simulink model "Experiment_AERO_pitch_channel"  (Simulink 8.9)
settings: Solver=ode4  StartTime=0.0  StopTime=100  FixedStep=0.001  RelTol=1e-3  EnableMultiTasking=on
InitFcn:
  | Parameters_and_initial_conditions
values from neighbouring files (symbols this model uses):
  A_p = [0 1 ... (first row only)    [Parameters_and_initial_conditions.m]
  B_p = [0 ... (first row only)    [Parameters_and_initial_conditions.m]
  C_p = [1 0;0 1]    [Parameters_and_initial_conditions.m]
  D_p = [0;0]    [Parameters_and_initial_conditions.m]
  Dp = 0.007768621416960    (= 0.00776862141696)    [Parameters_and_initial_conditions.m]
  Dp_static = Dp*0.05    (= 0.000388431070848)    [Parameters_and_initial_conditions.m]
  Dy = 0.0220    (= 0.022)    [Parameters_and_initial_conditions.m]
  G_bar_D = [(Jp*T^2) (T^2*Dp+2*Jp*T) (T^2*Ksp+2*T*Dp+T*k2+Jp) (2*T*Ksp+T*k1+Dp+k2) (Ksp+k1)]    [Parameters_and_initial_conditions.m]
  G_bar_N11 = [(Jp*T) (T*Dp+Jp) (T*Ksp+Dp+k2) Ksp]    [Parameters_and_initial_conditions.m]
  G_bar_N12 = [-k2]    [Parameters_and_initial_conditions.m]
  G_bar_N21 = [-k1 0]    [Parameters_and_initial_conditions.m]
  G_bar_N22 = [(Jp*T) (T*Dp+Jp) (T*Ksp+Dp) (Ksp+k1)]    [Parameters_and_initial_conditions.m]
  Invalid_T = 1    [Parameters_and_initial_conditions.m]
  Jp = J_body + 2*J_prop    (= 0.0218868648283)    [Parameters_and_initial_conditions.m]
  Jy = J_body + 2*J_prop + J_yoke    (= 0.0219920648283)    [Parameters_and_initial_conditions.m]
  k1 = 0.1    [Parameters_and_initial_conditions.m]
  k2 = 0.05    [Parameters_and_initial_conditions.m]
  Kpp = 9.971955650940002e-04    (= 0.000997195565094)    [Parameters_and_initial_conditions.m]
  Kpy = 0.0021    [Parameters_and_initial_conditions.m]
  Ksp = 0.071643279410402    (= 0.0716432794104)    [Parameters_and_initial_conditions.m]
  Kyp = -0.0027    [Parameters_and_initial_conditions.m]
  Kyy = 0.0022    [Parameters_and_initial_conditions.m]
  PitchAxisEnable = 1    [Parameters_and_initial_conditions.m]
  PitchMotorEnable = 1    [Parameters_and_initial_conditions.m]
  psi_dot_initial = 0.0    (= 0)    [Parameters_and_initial_conditions.m]
  psi_initial = 0.0    (= 0)    [Parameters_and_initial_conditions.m]
  T = 2    [Parameters_and_initial_conditions.m]
  theta_dot_initial = 0.0    (= 0)    [Parameters_and_initial_conditions.m]
  theta_initial = 0.0    (= 0)    [Parameters_and_initial_conditions.m]
  YawAxisEnable = 0    [Parameters_and_initial_conditions.m]
  YawMotorEnable = 0    [Parameters_and_initial_conditions.m]
undefined symbols (not defined in the file or in its folder): Continuous, Time
libraries: simulink_extras x11, quarc_library x9, ctrlSharedLib x1, quanser_aero x1
settings Model: Creator=MLevis  LastModifiedBy=fsc  SimulationMode=external  ExtModeTrigDuration=5000
settings SolverCC: PositivePriorityOrder=on
settings DataIOCC: SignalLoggingSaveFormat=Dataset
settings DebuggingCC: UnderspecifiedInitializationDetection=Simplified  MergeDetectMultiDrivingBlocksExec=error  SolverPrmCheckMsg=warning  FcnCallInpInsideContextMsg=error  StateNameClashWarn=none
settings RTWCC: SystemTargetFile=quarc_win64.tlc  TemplateMakefile=quarc_default_tmf  Description=QUARC Win64 Target
settings STFCustomTargetCC: TargetPreCompLibLocation=C:\PROGRA~3\QUARC\lib\2017a\win64\release  ConcurrentExecutionCompliant=on  GeneratePreprocessorConditionals=Disable all  SystemTargetFile=quarc_win64.tlc
settings GRTTargetCC: TargetPreCompLibLocation=C:\PROGRA~3\QUARC\lib\2017a\win64\release  ParMdlRefBuildCompliant=off  CompOptLevelCompliant=off  MatFileLogging=off  CPPClassGenCompliant=off  UseToolchainInfoCompliant=off  ExtMode=on  ExtModeMexFile=quarc_comm
settings ConfigComp: CovSFcnEnable=off

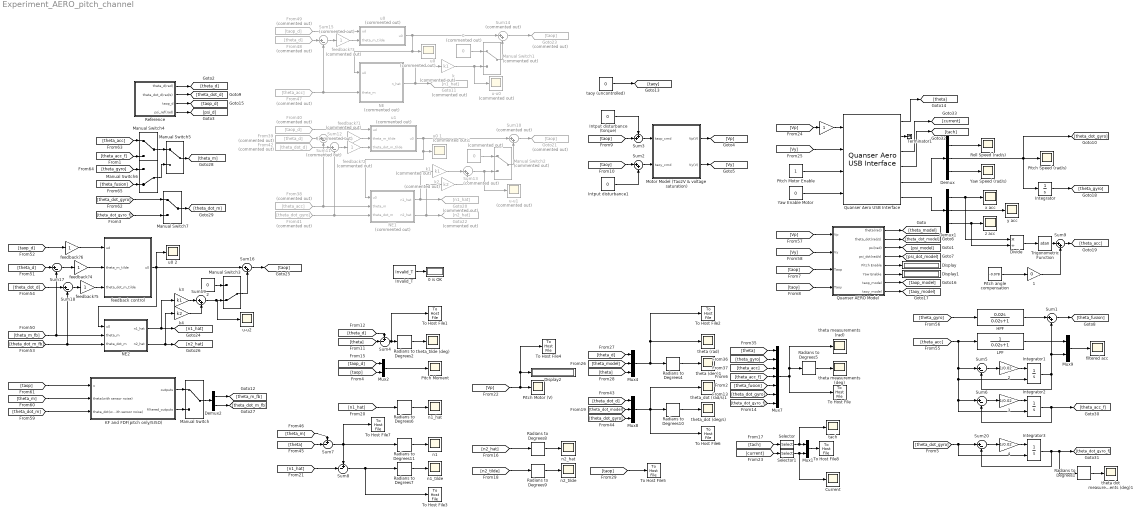
== system Experiment_AERO_pitch_channel ==
  " " : Gain
  " 1" : Gain  Gain=0
  " 2" : Gain  Gain=1/0.02
  " 3" : Gain  Gain=1/0.02
  " 4" : Gain  Gain=1/0.02
  " feedback?1" : Gain  Commented=on
  " feedback?2" : Gain  Commented=on
  " feedback?3" : Gain  Commented=on
  " feedback?4" : Gain
  " feedback?5" : Gain
  " feedback?6" : Gain
  0 : Constant  Commented=on  Value=0
  0 is OK : Display
  1 : Constant  Commented=on  Value=0
  2 : Constant  Value=0
  Current : Scope
  Demux : Demux  Outputs=3
  Demux1 : Demux  Outputs=3
  Demux2 : Demux  Outputs=2
  Display : Display
  Display1 : Display
  Display2 : Display
  Divide : Product  Inputs=*/
  From38 : From  Commented=on  GotoTag=theta_acc
  From39 : From  Commented=on  GotoTag=theta_d
  From40 : From  Commented=on  GotoTag=taop_d
  From41 : From  Commented=on  GotoTag=theta_dot_gyro
  From42 : From  Commented=on  GotoTag=theta_dot_d
  From47 : From  Commented=on  GotoTag=theta_acc
  From48 : From  Commented=on  GotoTag=theta_d
  From49 : From  Commented=on  GotoTag=taop_d
  Goto11 : Goto  Commented=on  GotoTag=n1_hat
  Goto20 : Goto  Commented=on  GotoTag=n1_hat
  Goto21 : Goto  Commented=on  GotoTag=taop
  Goto22 : Goto  Commented=on  GotoTag=n2_hat
  Goto23 : Goto  Commented=on  GotoTag=taop
  HPF : TransferFcn  Numerator=[0.02 0]  Denominator=[0.02 1]
  Integrator : Integrator
  Integrator1 : Integrator  InitialConditionSource=external
  Integrator2 : Integrator  InitialConditionSource=external
  Integrator3 : Integrator  InitialConditionSource=external
  Intput disturbance (torque) : Constant  Value=0
  Intput disturbance1 : Constant  Value=0
  Invalid_T : Constant  Value=Invalid_T
  KF and FDF(pitch only/SISO) : Subsystem
  LPF : TransferFcn  Denominator=[0.02 1]
  Manual Switch{,4..5,7} (4 alike) : ManualSwitch
  Manual Switch1 : ManualSwitch  Commented=on
  Manual Switch2 : ManualSwitch  Commented=on
  Manual Switch3 : ManualSwitch  CurrentSetting=0
  Manual Switch6 : ManualSwitch  CurrentSetting=0
  Motor Model (Tao2V & voltage saturation) : Subsystem
  Mux1 : Mux  Inputs=2
  Mux2 : Mux  Inputs=2
  Mux4 : Mux  Inputs=3
  Mux7 : Mux  Inputs=7
  Mux8 : Mux  Inputs=3
  Mux9 : Mux  Inputs=2
  NE : Subsystem  Commented=on
  NE1 : Subsystem  Commented=on
  NE2 : Subsystem
  Pitch Moment : Scope
  Pitch Motor (V) : Scope
  Pitch Motor Enable : Constant
  Pitch Speed (rad/s) : Scope
  Pitch angle compensation : Constant  Value=-0.078
  Quanser AERO Model : Subsystem
  Quanser Aero USB Interface : quanser_aero/Quanser Aero USB Interface
  Radians to Degrees{1..2,4..11} (10 alike) : simulink_extras/Transformations/Radians to Degrees
  Reference : Subsystem
  Roll Speed (rad/s) : Scope
  Selector : Selector  InputPortWidth=2  IndexOptions=Index vector (dialog)  Indices=[1]  OutputSizes=1
  Selector1 : Selector  InputPortWidth=2  IndexOptions=Index vector (dialog)  Indices=[1]  OutputSizes=1
  Sum{1..2,9,16,19} (5 alike) : Sum  Inputs=|++
  Sum10 : Sum  Commented=on  Inputs=|++
  Sum11 : Sum  Commented=on  Inputs=|+-
  Sum12 : Sum  Commented=on  Inputs=|+-
  Sum13 : Sum  Commented=on  Inputs=|++
  Sum14 : Sum  Commented=on  Inputs=|++
  Sum15 : Sum  Commented=on  Inputs=|+-
  Sum{5..6,17..18,20} (5 alike) : Sum  Inputs=|+-
  Sum3 : Sum  Inputs=++|
  Sum4 : Sum  Inputs=+-|
  Sum7 : Sum  Inputs=+-|
  Sum8 : Sum  Inputs=+-|
  Terminator1 : Terminator
  To Host File : quarc_library/Sinks/To Host/To Host File  file_name=Log_Sensor_Measurements.mat  variable_name=Log_Sensor_Measurements  decimation=1  sample_time=-1  file_format=MAT-file v.5  options=No header or footer  append=off  final_file_name=Log_Sensor_Measurements.mat  bitrate=2000000
  To Host File1 : quarc_library/Sinks/To Host/To Host File  file_name=Log_Tracking_Err.mat  variable_name=Log_Tracking_Err  decimation=1  sample_time=-1  file_format=MAT-file v.5  options=No header or footer  append=off  final_file_name=Log_Tracking_Err.mat  bitrate=2000000
  To Host File2 : quarc_library/Sinks/To Host/To Host File  file_name=Log_Theta_Response.mat  variable_name=Log_Theta_Response  decimation=1  sample_time=-1  file_format=MAT-file v.5  options=No header or footer  append=off  final_file_name=Log_Theta_Response.mat  bitrate=2000000
  To Host File3 : quarc_library/Sinks/To Host/To Host File  file_name=Log_Noise_Estimation_Err.mat  variable_name=Log_Noise_Estimation_Err  decimation=1  sample_time=-1  file_format=MAT-file v.5  options=No header or footer  append=off  final_file_name=Log_Noise_Estimation_Err.mat  bitrate=2000000
  To Host File4 : quarc_library/Sinks/To Host/To Host File  file_name=Log_Input_Voltage.mat  variable_name=Log_Input_Voltage  decimation=1  sample_time=-1  file_format=MAT-file v.5  options=No header or footer  append=off  final_file_name=Log_Input_Voltage.mat  bitrate=2000000
  To Host File5 : quarc_library/Sinks/To Host/To Host File  file_name=Log_Input_Torque.mat  variable_name=Log_Input_Torque  decimation=1  sample_time=-1  file_format=MAT-file v.5  options=No header or footer  append=off  final_file_name=Log_Input_Torque.mat  bitrate=2000000
  To Host File6 : quarc_library/Sinks/To Host/To Host File  file_name=Log_Theta_dot_Response.mat  variable_name=Log_Theta_dot_Response  decimation=1  sample_time=-1  file_format=MAT-file v.5  options=No header or footer  append=off  final_file_name=Log_Theta_dot_Response.mat  bitrate=2000000
  To Host File7 : quarc_library/Sinks/To Host/To Host File  file_name=Log_Noise.mat  variable_name=Log_Noise  decimation=1  sample_time=-1  file_format=MAT-file v.5  options=No header or footer  append=off  final_file_name=Log_Noise.mat  bitrate=2000000
  To Host File8 : quarc_library/Sinks/To Host/To Host File  file_name=Log_Tach_Current.mat  variable_name=Log_Tach_Current  decimation=1  sample_time=-1  file_format=MAT-file v.5  options=No header or footer  append=off  final_file_name=Log_Tach_Current.mat  bitrate=2000000
  Trigonometric Function : Trigonometry  Operator=atan
  Yaw Enable Motor : Constant  Value=0
  Yaw Speed (rad/s) : Scope
  feedback control : Subsystem
  filtered acc : Scope
  k : Gain  Commented=on  Gain=k1
  k1 : Gain  Commented=on  Gain=k1
  k2 : Gain  Commented=on  Gain=k2
  k3 : Gain  Gain=k1
  k4 : Gain  Gain=k2
  n1 : Scope
  n1_hat : Scope
  n1_tilde : Scope
  n2_hat : Scope
  n2_tilde : Scope
  tach : Scope
  taoy (uncontrolled) : Constant  Value=0
  theta (deg)1 : Scope
  theta (rad) : Scope
  theta dot measurements (deg)1 : Scope
  theta measurements (deg) : Scope
  theta measurements (rad) : Scope
  theta_dot (deg/s) : Scope
  theta_dot (rad/s)1 : Scope
  theta_tilde (deg) : Scope
  u-u0 : Scope  Commented=on
  u-u1 : Scope  Commented=on
  u-u2 : Scope
  u0 : Subsystem  Commented=on
  "u0 " : Scope  Commented=on
  u0 1 : Scope  Commented=on
  u0 2 : Scope
  u1 : Subsystem  Commented=on
  x acc : Scope
  y acc : Scope
  z acc : Scope
  wires:
  Quanser AERO Model/3(psi(rad)) -> [psi_model]
  Quanser AERO Model/1(theta(rad)) -> [theta_model]
  Reference/1(theta_d(rad)) -> [theta_d]
  Reference/4(psi_ref(rad)) -> [psi_d]
  Mux2/1 -> Pitch Moment/1
  Quanser AERO Model/2(theta_dot(rad/s)) -> [theta_dot_model]
  Quanser AERO Model/4(psi_dot(rad/s)) -> [psi_dot_model]
  Quanser AERO Model/5(Pitch Enable) -> Display/1
  Quanser AERO Model/6(Yaw Enable) -> Display1/1
  Motor Model (Tao2V & voltage saturation)/1(Vp(V)) -> [Vp]
  Motor Model (Tao2V & voltage saturation)/2(Vy(V)) -> [Vy]
  [taop] -> Sum3/2
  [taoy] -> Sum2/1
  Intput disturbance (torque)/1 -> Sum3/1
  Sum2/1 -> Motor Model (Tao2V & voltage saturation)/2(taoy_cmd)
  Sum3/1 -> Motor Model (Tao2V & voltage saturation)/1(taop_cmd)
  Intput disturbance1/1 -> Sum2/2
  [theta_d] -> Sum4/1
  [theta] -> Sum4/2
  Sum4/1 -> To Host File1/1, Radians to Degrees2/1
  Radians to Degrees2/1 -> theta_tilde (deg)/1
  Reference/2(theta_dot_d(rad/s)) -> [theta_dot_d]
  Reference/3(taop_d) -> [taop_d]
  [taop] -> Mux2/2
  [taop_d] -> Mux2/1
  Invalid_T/1 -> 0 is OK/1
  taoy (uncontrolled)/1 -> [taoy]
  [Vp] -> To Host File4/1, Display2/1, Pitch Motor (V)/1
  Quanser Aero USB Interface/5 -> Demux/1
  Yaw Enable Motor/1 -> Quanser Aero USB Interface/4
  Quanser Aero USB Interface/4 -> [tach]
  [Vp] -> " "/1
  Quanser Aero USB Interface/1 -> [theta]
  Demux/3 -> Yaw Speed (rad/s)/1
  Pitch Motor Enable/1 -> Quanser Aero USB Interface/3
  Quanser Aero USB Interface/3 -> [current]
  [Vy] -> Quanser Aero USB Interface/2
  Demux/1 -> Roll Speed (rad/s)/1
  Demux/2 -> [theta_dot_gyro], Integrator/1, Pitch Speed (rad/s)/1
  Quanser Aero USB Interface/2 -> Terminator1/1
  Quanser Aero USB Interface/6 -> Demux1/1
  " "/1 -> Quanser Aero USB Interface/1
  Radians to Degrees4/1 -> theta (deg)1/1
  [theta_model] -> Mux4/2
  [theta_d] -> Mux4/1
  [theta] -> Mux4/3
  Quanser AERO Model/7(taop_model) -> [taop_model]
  [taop] -> To Host File5/1
  Quanser AERO Model/8(taoy_model) -> [taoy_model]
  Integrator/1 -> [theta_gyro]
  [theta] -> Mux7/1
  Demux1/1 -> Divide/1, x acc/1
  Demux1/2 -> y acc/1
  Demux1/3 -> Divide/2, z acc/1
  Divide/1 -> Trigonometric Function/1
  Trigonometric Function/1 -> Sum9/1
  Sum9/1 -> [theta_acc]
  Pitch angle compensation/1 -> " 1"/1
  [theta_gyro] -> Mux7/2
  [theta_acc] -> Mux7/3
  Radians to Degrees5/1 -> theta measurements (deg)/1
  Manual Switch2/1 -> Sum10/2
  Sum11/1 -> " feedback?1"/1
  u1/1(u0) -> Sum10/1, NE1/1(u0), u0 1/1
  k1/1 -> Sum13/1
  NE1/1(n1_hat) -> Goto20/1, k1/1
  From39/1 -> Sum11/1
  Sum13/1 -> u-u1/1, Manual Switch2/2
  From40/1 -> u1/1(ud)
  From41/1 -> Sum12/2, NE1/3(theta_dot_m)
  k2/1 -> Sum13/2
  Sum12/1 -> " feedback?2"/1
  NE1/2(n2_hat) -> k2/1, Goto22/1
  Sum10/1 -> Goto21/1
  From38/1 -> Sum11/2, NE1/2(theta_m)
  1/1 -> Manual Switch2/1
  From42/1 -> Sum12/1
  " feedback?1"/1 -> u1/2(theta_m_tilde)
  " feedback?2"/1 -> u1/3(theta_dot_m_tilde)
  Sum8/1 -> To Host File3/1, Radians to Degrees7/1
  Radians to Degrees9/1 -> n2_tilde/1
  Radians to Degrees6/1 -> n1_hat/1
  [n2_tilde] -> Radians to Degrees9/1
  Radians to Degrees8/1 -> n2_hat/1
  [n2_hat] -> Radians to Degrees8/1
  [n1_hat] -> Radians to Degrees6/1
  Radians to Degrees7/1 -> n1_tilde/1
  Radians to Degrees10/1 -> theta_dot (deg/s)/1
  [theta_dot_model] -> Mux8/2
  Mux8/1 -> To Host File6/1, theta_dot (rad/s)1/1, Radians to Degrees10/1
  [theta_dot_gyro] -> Mux8/3
  [theta_dot_d] -> Mux8/1
  [theta_m] -> Sum7/1
  [theta] -> Sum7/2
  Sum7/1 -> To Host File7/1, Sum8/1, Radians to Degrees11/1
  [n1_hat] -> Sum8/2
  Radians to Degrees11/1 -> n1/1
  " 1"/1 -> Sum9/2
  0/1 -> Manual Switch1/1
  From48/1 -> Sum15/1
  Sum15/1 -> " feedback?3"/1
  From49/1 -> u0/1(ud)
  Manual Switch1/1 -> Sum14/2
  Sum14/1 -> Goto23/1
  NE/1(n_hat) -> Goto11/1, k/1
  k/1 -> u-u0/1, Manual Switch1/2
  From47/1 -> Sum15/2, NE/2(theta_m)
  u0/1(u0) -> "u0 "/1, NE/1(u0), Sum14/1
  " feedback?3"/1 -> u0/2(theta_m_tilde)
  Sum16/1 -> [taop]
  [taop_d] -> " feedback?6"/1
  [theta_dot_m_fb] -> Sum18/2, NE2/3(theta_dot_m)
  [theta_m_fb] -> Sum17/2, NE2/2(theta_m)
  Manual Switch3/1 -> Sum16/2
  " feedback?5"/1 -> feedback control/3(theta_dot_m_tilde)
  Sum19/1 -> u-u2/1, Manual Switch3/2
  [theta_dot_d] -> Sum18/1
  Sum18/1 -> " feedback?5"/1
  feedback control/1(u0) -> NE2/1(u0), u0 2/1, Sum16/1
  [theta_d] -> Sum17/1
  NE2/1(n1_hat) -> [n1_hat], k3/1
  " feedback?4"/1 -> feedback control/2(theta_m_tilde)
  k3/1 -> Sum19/1
  NE2/2(n2_hat) -> k4/1, [n2_hat]
  2/1 -> Manual Switch3/1
  Sum17/1 -> " feedback?4"/1
  k4/1 -> Sum19/2
  [theta_gyro] -> HPF/1
  HPF/1 -> Sum1/1
  LPF/1 -> Mux9/1
  Sum1/1 -> [theta_fusion]
  [theta_acc_f] -> Mux7/4
  Mux7/1 -> theta measurements (rad)/1, Radians to Degrees5/1, To Host File/1
  Integrator1/1 -> Sum5/2, Sum1/2, Mux9/2
  Sum5/1 -> " 2"/1
  " 2"/1 -> Integrator1/1
  Mux9/1 -> filtered acc/1
  [taop] -> Quanser AERO Model/3(Taop)
  [taoy] -> Quanser AERO Model/4(Taoy)
  [Vp] -> Quanser AERO Model/1(Vp)
  [Vy] -> Quanser AERO Model/2(Vy)
  " feedback?6"/1 -> feedback control/1(ud)
  [theta_dot_m] -> KF and FDF(pitch only/SISO)/3(theta_dot(with sensor noise))
  Demux2/2 -> [theta_dot_m_fb]
  Demux2/1 -> [theta_m_fb]
  [taop] -> KF and FDF(pitch only/SISO)/1(u)
  KF and FDF(pitch only/SISO)/2(filtered_outputs) -> Manual Switch/2
  KF and FDF(pitch only/SISO)/1(outputs) -> Manual Switch/1
  Manual Switch/1 -> Demux2/1
  Manual Switch7/1 -> [theta_dot_m]
  [theta_acc] -> Manual Switch4/1
  [theta_gyro] -> Manual Switch6/1
  Manual Switch4/1 -> Manual Switch5/1
  Manual Switch5/1 -> [theta_m]
  [theta_fusion] -> Manual Switch6/2
  [theta_m] -> KF and FDF(pitch only/SISO)/2(theta(with sensor noise))
  Mux4/1 -> To Host File2/1, theta (rad)/1, Radians to Degrees4/1
  [theta_acc_f] -> Manual Switch4/2
  Manual Switch6/1 -> Manual Switch5/2
  Integrator2/1 -> Sum6/2, [theta_acc_f]
  " 3"/1 -> Integrator2/1
  Sum6/1 -> " 3"/1
  [theta_acc] -> Sum6/1, Integrator2/2, Integrator1/2, Sum5/1, LPF/1
  [theta_fusion] -> Mux7/5
  [theta_dot_gyro] -> Manual Switch7/1
  [theta_dot_gyro_f] -> Manual Switch7/2
  [theta_dot_gyro] -> Integrator3/2, Sum20/1
  Sum20/1 -> " 4"/1
  " 4"/1 -> Integrator3/1
  Integrator3/1 -> Radians to Degrees1/1, [theta_dot_gyro_f], Sum20/2
  Radians to Degrees1/1 -> theta dot measurements (deg)1/1
  [theta_dot_gyro] -> Mux7/6
  [theta_dot_gyro_f] -> Mux7/7
  [tach] -> Selector/1
  Mux1/1 -> To Host File8/1
  [current] -> Selector1/1
  Selector/1 -> tach/1, Mux1/1
  Selector1/1 -> Current/1, Mux1/2

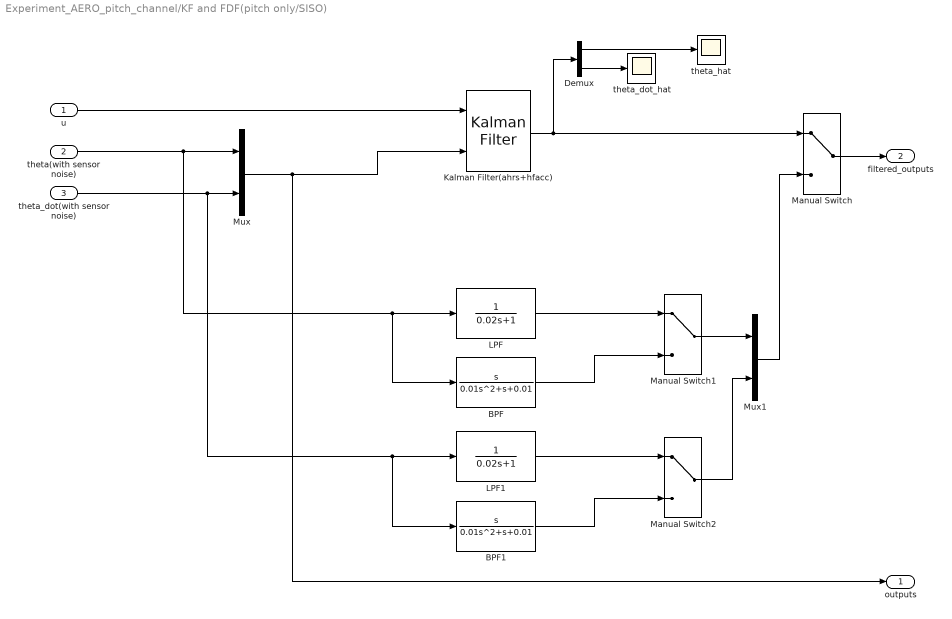
== system Experiment_AERO_pitch_channel/KF and FDF(pitch only/SISO) ==
  u : Inport
  theta(with sensor noise) : Inport  Port=2
  theta_dot(with sensor noise) : Inport  Port=3
  BPF : TransferFcn  Numerator=[1 0]  Denominator=[0.01 1 0.01]
  BPF1 : TransferFcn  Numerator=[1 0]  Denominator=[0.01 1 0.01]
  Demux : Demux  Outputs=2
  Kalman Filter(ahrs+hfacc) : ctrlSharedLib/Kalman Filter  TimeDomain=Continuous-Time  UseCurrentEstimator=on  ModelSource=Individual A, B, C, D matrices  ModelSourceVariable=ss(0.95,1,1,0,1)  A=A_p  B=B_p  C=C_p  D=D_p  NumberOfStates=1  NumberOfInputs=1  NumberOfOutputs=1  InitialEstimateSource=Dialog  X0=[theta_initial; theta_dot_initial]  P0=10  UseK=off  UseGH=off  NumberOfProcessNoiseInputs=1  G=1  TimeInvariantG=on  H=0  TimeInvariantH=on  Q=0.05*[1 0; 0 1]  TimeInvariantQ=on  R=[0.1 0.1]  TimeInvariantR=on  N=0  TimeInvariantN=on  AddInputPort=on  AddEnablePort=off  ExternalReset=none  OutputEstimatedY=off  OutputP=off  Ts=-1
  LPF : TransferFcn  Denominator=[0.02 1]
  LPF1 : TransferFcn  Denominator=[0.02 1]
  Manual Switch : ManualSwitch
  Manual Switch1 : ManualSwitch
  Manual Switch2 : ManualSwitch
  Mux : Mux  Inputs=2
  Mux1 : Mux  Inputs=2
  theta_dot_hat : Scope
  theta_hat : Scope
  outputs : Outport
  filtered_outputs : Outport  Port=2
  wires:
  Manual Switch/1 -> filtered_outputs/1
  u/1 -> Kalman Filter(ahrs+hfacc)/1
  Kalman Filter(ahrs+hfacc)/1 -> Demux/1, Manual Switch/1
  LPF/1 -> Manual Switch1/1
  theta(with sensor noise)/1 -> BPF/1, LPF/1, Mux/1
  BPF/1 -> Manual Switch1/2
  Demux/1 -> theta_hat/1
  Demux/2 -> theta_dot_hat/1
  Mux/1 -> outputs/1, Kalman Filter(ahrs+hfacc)/2
  LPF1/1 -> Manual Switch2/1
  theta_dot(with sensor noise)/1 -> LPF1/1, BPF1/1, Mux/2
  BPF1/1 -> Manual Switch2/2
  Manual Switch1/1 -> Mux1/1
  Manual Switch2/1 -> Mux1/2
  Mux1/1 -> Manual Switch/2

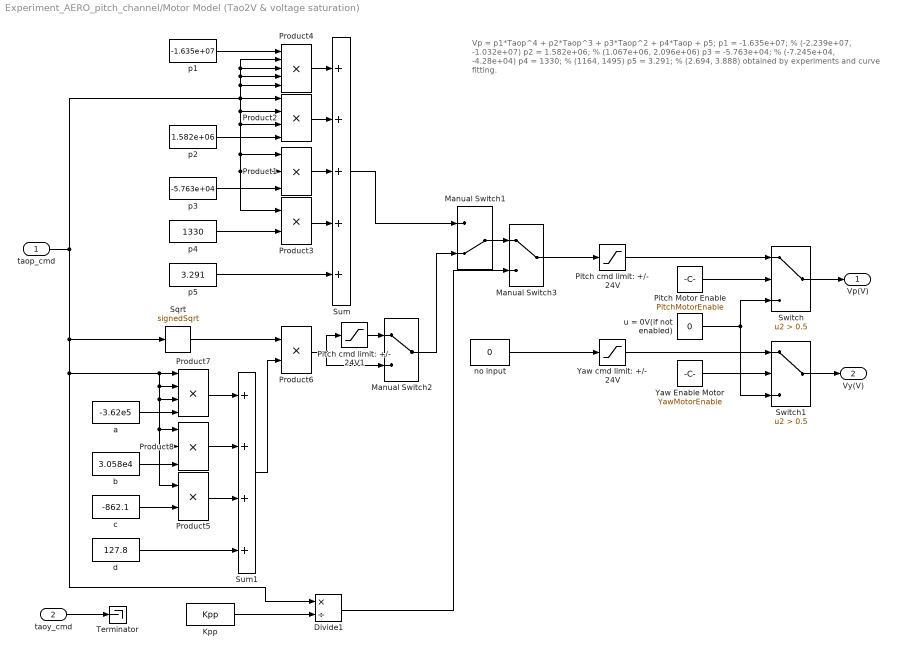
== system Experiment_AERO_pitch_channel/Motor Model (Tao2V & voltage saturation) ==
  note: Vp = p1*Taop^4 + p2*Taop^3 + p3*Taop^2 + p4*Taop + p5;
      | p1 = -1.635e+07; % (-2.239e+07, -1.032e+07)
      | p2 = 1.582e+06; % (1.067e+06, 2.096e+06)
      | p3 = -5.763e+04; % (-7.245e+04, -4.28e+04)
      | p4 = 1330; % (1164, 1495)
      | p5 = 3.291; % (2.694, 3.888)
      |
      | obtained by experiments and curve fitting.
  taop_cmd : Inport
  taoy_cmd : Inport  Port=2
  Divide1 : Product  Inputs=*/
  Kpp : Constant  Value=Kpp
  Manual Switch1 : ManualSwitch  CurrentSetting=0
  Manual Switch2 : ManualSwitch
  Manual Switch3 : ManualSwitch
  Pitch Motor Enable : Constant  Value=PitchMotorEnable
  Pitch cmd limit: +/- 24V : Saturate  UpperLimit=24  LowerLimit=-24
  Pitch cmd limit: +/- 24V1 : Saturate  UpperLimit=24  LowerLimit=0
  Product1 : Product  Inputs=3
  Product2 : Product  Inputs=4
  Product3 : Product
  Product4 : Product  Inputs=5
  Product5 : Product
  Product6 : Product
  Product7 : Product  Inputs=4
  Product8 : Product  Inputs=3
  Sqrt : Sqrt  Operator=signedSqrt  SaturateOnIntegerOverflow=on
  Sum : Sum  Inputs=+++++
  Sum1 : Sum  Inputs=++++
  Switch : Switch  Criteria=u2 > Threshold  Threshold=0.5
  Switch1 : Switch  Criteria=u2 > Threshold  Threshold=0.5
  Terminator : Terminator
  Yaw Enable Motor : Constant  Value=YawMotorEnable
  Yaw cmd limit: +/- 24V : Saturate  UpperLimit=24  LowerLimit=-24
  a : Constant  Value=-3.62e5
  b : Constant  Value=3.058e4
  c : Constant  Value=-862.1
  d : Constant  Value=127.8
  no input : Constant  Value=0
  p1 : Constant  Value=-1.635e+07
  p2 : Constant  Value=1.582e+06
  p3 : Constant  Value=-5.763e+04
  p4 : Constant  Value=1330
  p5 : Constant  Value=3.291
  u = 0V(if not enabled) : Constant  Value=0
  Vp(V) : Outport
  Vy(V) : Outport  Port=2
  wires:
  Pitch Motor Enable/1 -> Switch/2
  Yaw Enable Motor/1 -> Switch1/2
  Switch/1 -> Vp(V)/1
  Switch1/1 -> Vy(V)/1
  Yaw cmd limit: +/- 24V/1 -> Switch1/1
  Pitch cmd limit: +/- 24V/1 -> Switch/1
  u = 0V(if not enabled)/1 -> Switch1/3, Switch/3
  taoy_cmd/1 -> Terminator/1
  p2/1 -> Product2/4
  no input/1 -> Yaw cmd limit: +/- 24V/1
  Product2/1 -> Sum/2
  p3/1 -> Product1/3
  p4/1 -> Product3/2
  Kpp/1 -> Divide1/2
  Product1/1 -> Sum/3
  Product3/1 -> Sum/4
  p5/1 -> Sum/5
  Sum/1 -> Manual Switch1/1
  Product4/1 -> Sum/1
  p1/1 -> Product4/1
  Manual Switch3/1 -> Pitch cmd limit: +/- 24V/1
  a/1 -> Product7/4
  b/1 -> Product8/3
  Sum1/1 -> Product6/2
  Sqrt/1 -> Product6/1
  Product6/1 -> Pitch cmd limit: +/- 24V1/1, Manual Switch2/2
  Manual Switch1/1 -> Manual Switch3/1
  Divide1/1 -> Manual Switch3/2
  d/1 -> Sum1/4
  Product7/1 -> Sum1/1
  Product8/1 -> Sum1/2
  Product5/1 -> Sum1/3
  c/1 -> Product5/2
  taop_cmd/1 -> Sqrt/1, Divide1/1, Product7/1, Product7/2, Product7/3, Product8/1, Product8/2, Product5/1, Product4/5, Product4/4, Product4/3, Product4/2, Product2/1, Product3/1, Product1/2, Product1/1, Product2/3, Product2/2
  Pitch cmd limit: +/- 24V1/1 -> Manual Switch2/1
  Manual Switch2/1 -> Manual Switch1/2

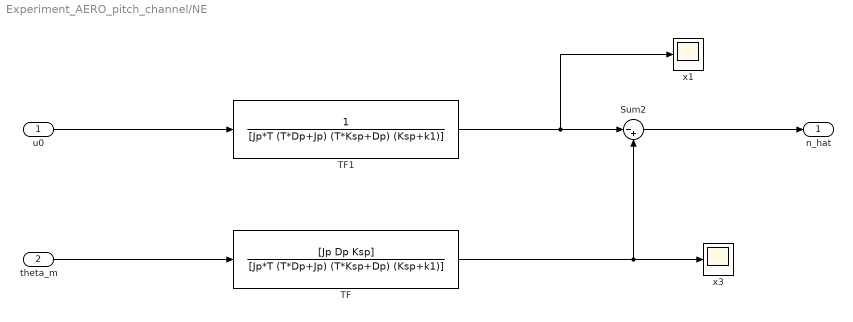
== system Experiment_AERO_pitch_channel/NE ==
  u0 : Inport
  theta_m : Inport  Port=2
  Sum2 : Sum  Inputs=|-+
  TF : TransferFcn  Numerator=[Jp Dp Ksp]  Denominator=[Jp*T (T*Dp+Jp) (T*Ksp+Dp) (Ksp+k1)]
  TF1 : TransferFcn  Denominator=[Jp*T (T*Dp+Jp) (T*Ksp+Dp) (Ksp+k1)]
  x1 : Scope
  x3 : Scope
  n_hat : Outport
  wires:
  theta_m/1 -> TF/1
  Sum2/1 -> n_hat/1
  TF/1 -> Sum2/2, x3/1
  u0/1 -> TF1/1
  TF1/1 -> x1/1, Sum2/1

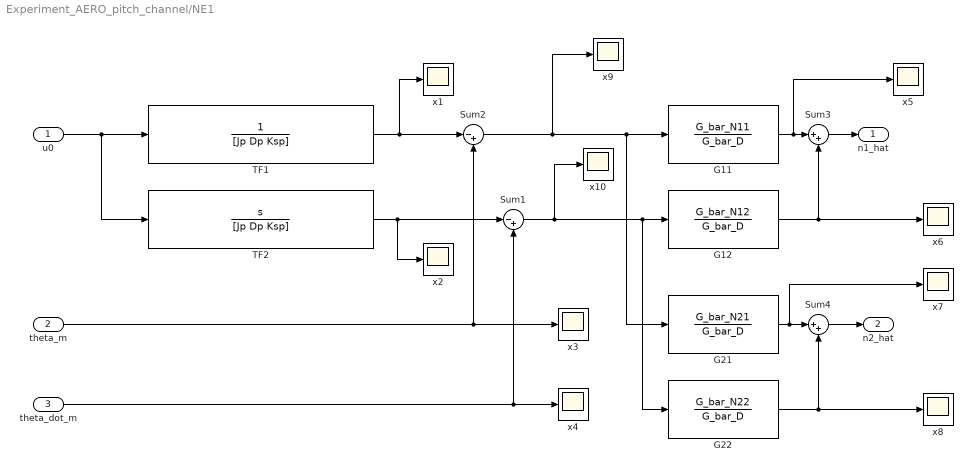
== system Experiment_AERO_pitch_channel/NE1 ==
  u0 : Inport
  theta_m : Inport  Port=2
  theta_dot_m : Inport  Port=3
  G11 : TransferFcn  Numerator=G_bar_N11  Denominator=G_bar_D
  G12 : TransferFcn  Numerator=G_bar_N12  Denominator=G_bar_D
  G21 : TransferFcn  Numerator=G_bar_N21  Denominator=G_bar_D
  G22 : TransferFcn  Numerator=G_bar_N22  Denominator=G_bar_D
  Sum1 : Sum  Inputs=|-+
  Sum2 : Sum  Inputs=|-+
  Sum3 : Sum  Inputs=|++
  Sum4 : Sum  Inputs=|++
  TF1 : TransferFcn  Denominator=[Jp Dp Ksp]
  TF2 : TransferFcn  Numerator=[1 0]  Denominator=[Jp Dp Ksp]
  x{1..10} (10 alike) : Scope
  n1_hat : Outport
  n2_hat : Outport  Port=2
  wires:
  Sum2/1 -> x9/1, G21/1, G11/1
  theta_m/1 -> Sum2/2, x3/1
  u0/1 -> TF2/1, TF1/1
  TF1/1 -> Sum2/1, x1/1
  TF2/1 -> x2/1, Sum1/1
  theta_dot_m/1 -> x4/1, Sum1/2
  Sum1/1 -> x10/1, G22/1, G12/1
  G12/1 -> x6/1, Sum3/2
  G11/1 -> x5/1, Sum3/1
  Sum3/1 -> n1_hat/1
  G22/1 -> x8/1, Sum4/2
  G21/1 -> x7/1, Sum4/1
  Sum4/1 -> n2_hat/1

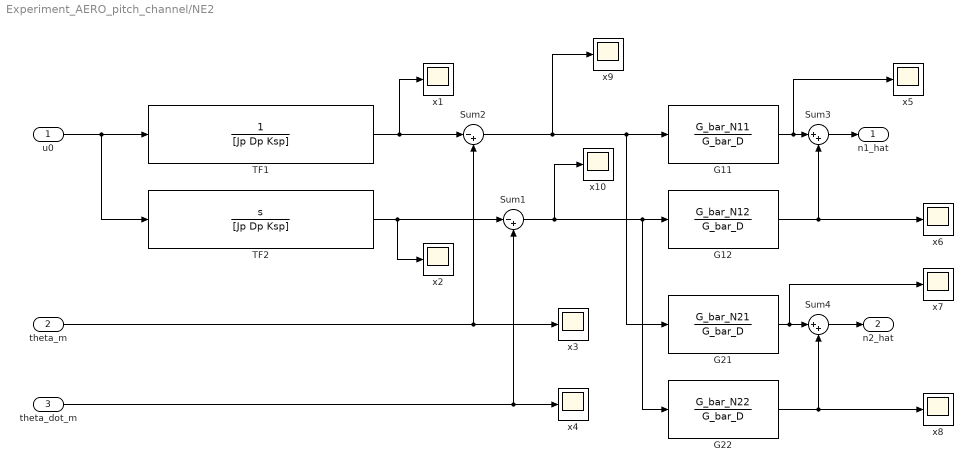
== system Experiment_AERO_pitch_channel/NE2 ==
  u0 : Inport
  theta_m : Inport  Port=2
  theta_dot_m : Inport  Port=3
  G11 : TransferFcn  Numerator=G_bar_N11  Denominator=G_bar_D
  G12 : TransferFcn  Numerator=G_bar_N12  Denominator=G_bar_D
  G21 : TransferFcn  Numerator=G_bar_N21  Denominator=G_bar_D
  G22 : TransferFcn  Numerator=G_bar_N22  Denominator=G_bar_D
  Sum1 : Sum  Inputs=|-+
  Sum2 : Sum  Inputs=|-+
  Sum3 : Sum  Inputs=|++
  Sum4 : Sum  Inputs=|++
  TF1 : TransferFcn  Denominator=[Jp Dp Ksp]
  TF2 : TransferFcn  Numerator=[1 0]  Denominator=[Jp Dp Ksp]
  x{1..10} (10 alike) : Scope
  n1_hat : Outport
  n2_hat : Outport  Port=2
  wires:
  Sum2/1 -> x9/1, G21/1, G11/1
  theta_m/1 -> Sum2/2, x3/1
  u0/1 -> TF2/1, TF1/1
  TF1/1 -> Sum2/1, x1/1
  TF2/1 -> x2/1, Sum1/1
  theta_dot_m/1 -> x4/1, Sum1/2
  Sum1/1 -> x10/1, G22/1, G12/1
  G12/1 -> x6/1, Sum3/2
  G11/1 -> x5/1, Sum3/1
  Sum3/1 -> n1_hat/1
  G22/1 -> x8/1, Sum4/2
  G21/1 -> x7/1, Sum4/1
  Sum4/1 -> n2_hat/1

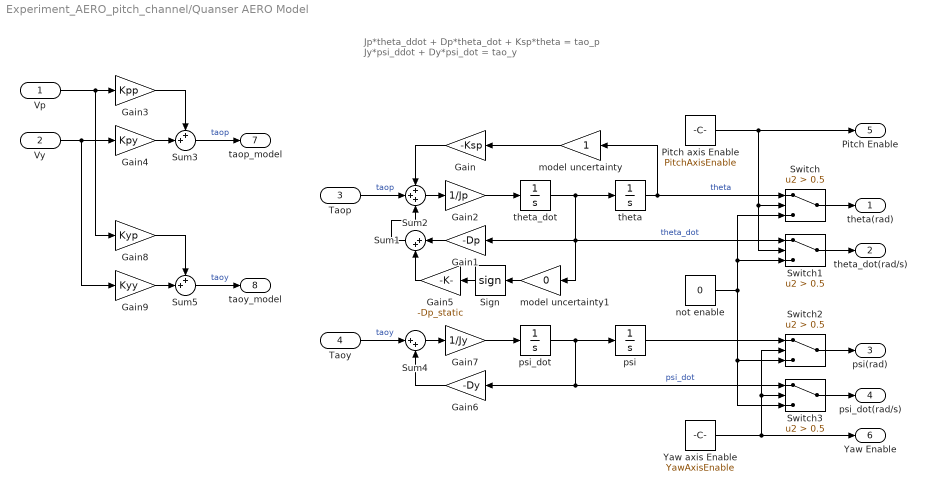
== system Experiment_AERO_pitch_channel/Quanser AERO Model ==
  note: Jp*theta_ddot + Dp*theta_dot + Ksp*theta = tao_p
      | Jy*psi_ddot + Dy*psi_dot = tao_y
  Vp : Inport
  Vy : Inport  Port=2
  Taop : Inport  Port=3
  Taoy : Inport  Port=4
  Gain : Gain  Gain=-Ksp
  Gain1 : Gain  Gain=-Dp
  Gain2 : Gain  Gain=1/Jp
  Gain3 : Gain  Gain=Kpp
  Gain4 : Gain  Gain=Kpy
  Gain5 : Gain  Gain=-Dp_static
  Gain6 : Gain  Gain=-Dy
  Gain7 : Gain  Gain=1/Jy
  Gain8 : Gain  Gain=Kyp
  Gain9 : Gain  Gain=Kyy
  Pitch axis Enable : Constant  Value=PitchAxisEnable
  Sign : Signum
  Sum1 : Sum  Inputs=|++
  Sum2 : Sum  Inputs=+++
  Sum3 : Sum  Inputs=++|
  Sum4 : Sum  Inputs=|++
  Sum5 : Sum  Inputs=++|
  Switch{,1..3} (4 alike) : Switch  Criteria=u2 > Threshold  Threshold=0.5
  Yaw axis Enable : Constant  Value=YawAxisEnable
  model uncertainty : Gain
  model uncertainty1 : Gain  Gain=0
  not enable : Constant  Value=0
  psi : Integrator  InitialCondition=psi_initial
  psi_dot : Integrator  InitialCondition=psi_dot_initial
  theta : Integrator  InitialCondition=theta_initial
  theta_dot : Integrator  InitialCondition=theta_dot_initial
  theta(rad) : Outport
  theta_dot(rad/s) : Outport  Port=2
  psi(rad) : Outport  Port=3
  psi_dot(rad/s) : Outport  Port=4
  Pitch Enable : Outport  Port=5
  Yaw Enable : Outport  Port=6
  taop_model : Outport  Port=7
  taoy_model : Outport  Port=8
  wires:
  theta_dot/1 -> model uncertainty1/1, Gain1/1, Switch1/1, theta/1  "theta_dot"
  theta/1 -> Switch/1, model uncertainty/1  "theta"
  Taop/1 -> Sum2/2  "taop"
  Gain/1 -> Sum2/1
  Gain1/1 -> Sum1/1
  Sum2/1 -> Gain2/1
  Gain2/1 -> theta_dot/1
  Gain3/1 -> Sum3/1
  Gain4/1 -> Sum3/2
  psi_dot/1 -> psi/1, Gain6/1, Switch3/1  "psi_dot"
  psi/1 -> Switch2/1
  Taoy/1 -> Sum4/1  "taoy"
  Sum4/1 -> Gain7/1
  Gain7/1 -> psi_dot/1
  Gain8/1 -> Sum5/1
  Gain9/1 -> Sum5/2
  Vp/1 -> Gain8/1, Gain3/1
  Vy/1 -> Gain9/1, Gain4/1
  Gain6/1 -> Sum4/2
  Pitch axis Enable/1 -> Pitch Enable/1, Switch1/2, Switch/2
  Switch/1 -> theta(rad)/1
  Switch1/1 -> theta_dot(rad/s)/1
  not enable/1 -> Switch1/3, Switch/3, Switch3/3, Switch2/3
  Switch2/1 -> psi(rad)/1
  Switch3/1 -> psi_dot(rad/s)/1
  Yaw axis Enable/1 -> Yaw Enable/1, Switch2/2, Switch3/2
  model uncertainty/1 -> Gain/1
  Sum1/1 -> Sum2/3
  Gain5/1 -> Sum1/2
  Sign/1 -> Gain5/1
  model uncertainty1/1 -> Sign/1
  Sum3/1 -> taop_model/1  "taop"
  Sum5/1 -> taoy_model/1  "taoy"

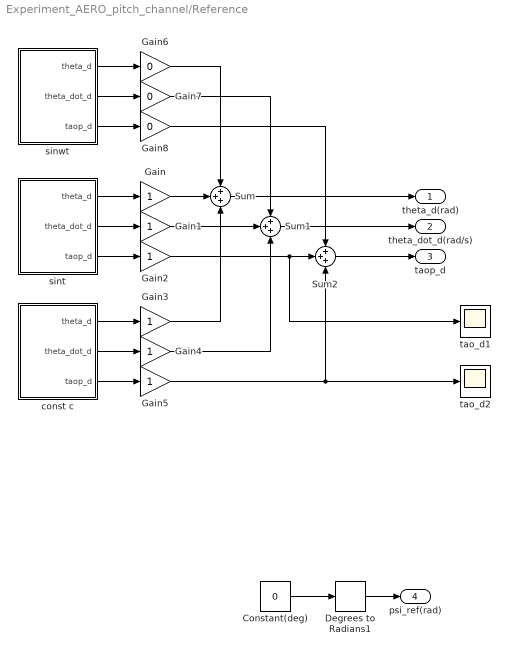
== system Experiment_AERO_pitch_channel/Reference ==
  Constant(deg) : Constant  Value=0
  Degrees to Radians1 : simulink_extras/Transformations/Degrees to Radians
  Gain{,1..5} (6 alike) : Gain
  Gain6 : Gain  Gain=0
  Gain7 : Gain  Gain=0
  Gain8 : Gain  Gain=0
  Sum : Sum  Inputs=+++
  Sum1 : Sum  Inputs=+++
  Sum2 : Sum  Inputs=+++
  const c : Subsystem
  sint : Subsystem
  sinwt : Subsystem
  tao_d1 : Scope
  tao_d2 : Scope
  theta_d(rad) : Outport
  theta_dot_d(rad/s) : Outport  Port=2
  taop_d : Outport  Port=3
  psi_ref(rad) : Outport  Port=4
  wires:
  Degrees to Radians1/1 -> psi_ref(rad)/1
  Constant(deg)/1 -> Degrees to Radians1/1
  Sum1/1 -> theta_dot_d(rad/s)/1
  Sum2/1 -> taop_d/1
  Sum/1 -> theta_d(rad)/1
  sint/1(theta_d) -> Gain/1
  const c/1(theta_d) -> Gain3/1
  sint/2(theta_dot_d) -> Gain1/1
  const c/2(theta_dot_d) -> Gain4/1
  sint/3(taop_d) -> Gain2/1
  const c/3(taop_d) -> Gain5/1
  Gain/1 -> Sum/2
  Gain1/1 -> Sum1/2
  Gain2/1 -> Sum2/2, tao_d1/1
  Gain3/1 -> Sum/3
  Gain4/1 -> Sum1/3
  Gain5/1 -> Sum2/3, tao_d2/1
  sinwt/3(taop_d) -> Gain8/1
  sinwt/2(theta_dot_d) -> Gain7/1
  sinwt/1(theta_d) -> Gain6/1
  Gain8/1 -> Sum2/1
  Gain7/1 -> Sum1/1
  Gain6/1 -> Sum/1

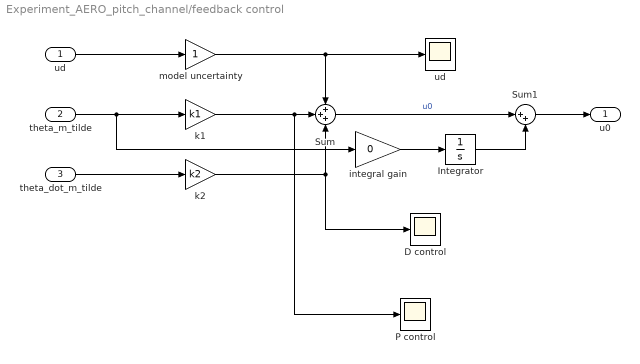
== system Experiment_AERO_pitch_channel/feedback control ==
  ud : Inport
  theta_m_tilde : Inport  Port=2
  theta_dot_m_tilde : Inport  Port=3
  D control : Scope
  Integrator : Integrator
  P control : Scope
  Sum : Sum  Inputs=+++
  Sum1 : Sum  Inputs=|++
  integral gain : Gain  Gain=0
  k1 : Gain  Gain=k1
  k2 : Gain  Gain=k2
  model uncertainty : Gain
  "ud " : Scope
  u0 : Outport
  wires:
  ud/1 -> model uncertainty/1
  theta_m_tilde/1 -> integral gain/1, k1/1
  k1/1 -> P control/1, Sum/2
  Sum/1 -> Sum1/1  "u0"
  theta_dot_m_tilde/1 -> k2/1
  k2/1 -> D control/1, Sum/3
  Sum1/1 -> u0/1
  Integrator/1 -> Sum1/2
  integral gain/1 -> Integrator/1
  model uncertainty/1 -> "ud "/1, Sum/1

== system Experiment_AERO_pitch_channel/u0 ==
  ud : Inport
  theta_m_tilde : Inport  Port=2
  Sum : Sum  Inputs=+++
  k : Gain  Gain=k1
  "ud " : Scope
  ud 1 : Scope
  u0 : Outport
  wires:
  ud/1 -> "ud "/1, Sum/1
  theta_m_tilde/1 -> k/1
  k/1 -> ud 1/1, Sum/2
  Sum/1 -> u0/1  "u0"

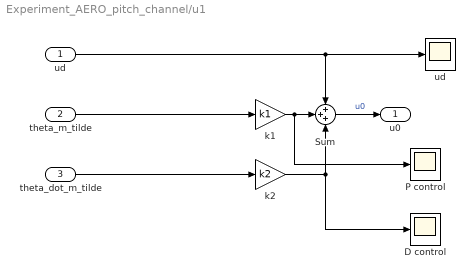
== system Experiment_AERO_pitch_channel/u1 ==
  ud : Inport
  theta_m_tilde : Inport  Port=2
  theta_dot_m_tilde : Inport  Port=3
  D control : Scope
  P control : Scope
  Sum : Sum  Inputs=+++
  k1 : Gain  Gain=k1
  k2 : Gain  Gain=k2
  "ud " : Scope
  u0 : Outport
  wires:
  ud/1 -> "ud "/1, Sum/1
  theta_m_tilde/1 -> k1/1
  k1/1 -> P control/1, Sum/2
  Sum/1 -> u0/1  "u0"
  theta_dot_m_tilde/1 -> k2/1
  k2/1 -> D control/1, Sum/3

== system Experiment_AERO_pitch_channel/Reference/const c ==
  Constant1 : Constant  Value=0
  Ksp : Gain  Gain=Ksp
  c : Constant  Value=0.2
  theta_d : Outport
  theta_dot_d : Outport  Port=2
  taop_d : Outport  Port=3
  wires:
  Ksp/1 -> taop_d/1
  c/1 -> theta_d/1, Ksp/1  "ud"
  Constant1/1 -> theta_dot_d/1

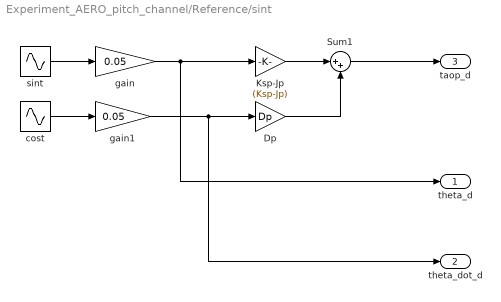
== system Experiment_AERO_pitch_channel/Reference/sint ==
  Dp : Gain  Gain=Dp
  Ksp-Jp : Gain  Gain=(Ksp-Jp)
  Sum1 : Sum  Inputs=|++
  cost : Sin  Phase=pi/2  SampleTime=0
  gain : Gain  Gain=0.05
  gain1 : Gain  Gain=0.05
  sint : Sin  SampleTime=0
  theta_d : Outport
  theta_dot_d : Outport  Port=2
  taop_d : Outport  Port=3
  wires:
  Dp/1 -> Sum1/2
  Ksp-Jp/1 -> Sum1/1
  sint/1 -> gain/1
  cost/1 -> gain1/1
  gain/1 -> theta_d/1, Ksp-Jp/1
  gain1/1 -> theta_dot_d/1, Dp/1
  Sum1/1 -> taop_d/1

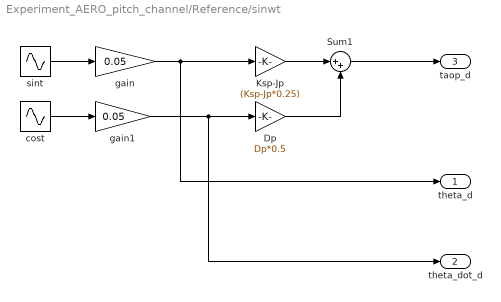
== system Experiment_AERO_pitch_channel/Reference/sinwt ==
  Dp : Gain  Gain=Dp*0.5
  Ksp-Jp : Gain  Gain=(Ksp-Jp*0.25)
  Sum1 : Sum  Inputs=|++
  cost : Sin  Frequency=0.5  Phase=pi/2  SampleTime=0
  gain : Gain  Gain=0.05
  gain1 : Gain  Gain=0.05
  sint : Sin  Frequency=0.5  SampleTime=0
  theta_d : Outport
  theta_dot_d : Outport  Port=2
  taop_d : Outport  Port=3
  wires:
  Sum1/1 -> taop_d/1
  gain1/1 -> Dp/1, theta_dot_d/1
  gain/1 -> Ksp-Jp/1, theta_d/1
  cost/1 -> gain1/1
  sint/1 -> gain/1
  Ksp-Jp/1 -> Sum1/1
  Dp/1 -> Sum1/2
